simulink model "new_my_brake_system"  (R2024a)
settings: Solver=ode45  StartTime=0  StopTime=2000  FixedStep=.001  RelTol=1e-3  EnableMultiTasking=on
model workspace (MAT data in the model file):
  J = 0.226199211484
  Kt = 174.53
  Ts_verif : Simulink.Parameter (value not decoded)
  angle_init = 15
  angle_open = 85
  c = 8.89069171842
  fall_end_angle : Simulink.Parameter (value not decoded)
  fall_start_angle : Simulink.Parameter (value not decoded)
  input_delay = 0.00986306560803
  k = 19.1559540807
  rise_end_angle : Simulink.Parameter (value not decoded)
  rise_start_angle : Simulink.Parameter (value not decoded)
  vv_fall_time_max : Simulink.Parameter (value not decoded)
  vv_fall_time_min : Simulink.Parameter (value not decoded)
  vv_rise_time_max : Simulink.Parameter (value not decoded)
  vv_rise_time_min : Simulink.Parameter (value not decoded)
(part 2 of 2)

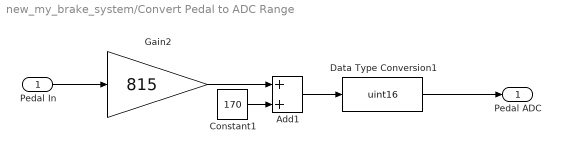
== system new_my_brake_system/Convert Pedal to ADC Range ==
  Pedal In : Inport
  Add1 : Sum
  Constant1 : Constant  Value=170
  Data Type Conversion1 : DataTypeConversion  OutDataTypeStr=uint16  SaturateOnIntegerOverflow=off  RndMeth=Floor
  Gain2 : Gain  Gain=815
  Pedal ADC : Outport  VectorParamsAs1DForOutWhenUnconnected=off
  wires:
  Gain2/1 -> Add1/1
  Constant1/1 -> Add1/2
  Data Type Conversion1/1 -> Pedal ADC/1
  Add1/1 -> Data Type Conversion1/1
  Pedal In/1 -> Gain2/1

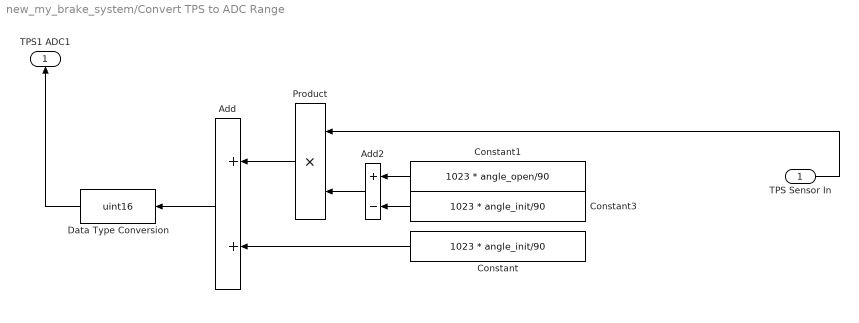
== system new_my_brake_system/Convert TPS to ADC Range ==
  TPS Sensor In : Inport
  Add : Sum
  Add2 : Sum  Inputs=+-
  Constant : Constant  Value=1023 * angle_init/90
  Constant1 : Constant  Value=1023 * angle_open/90
  Constant3 : Constant  Value=1023 * angle_init/90
  Data Type Conversion : DataTypeConversion  OutDataTypeStr=uint16  SaturateOnIntegerOverflow=off  RndMeth=Floor
  Product : Product
  TPS1 ADC1 : Outport  VectorParamsAs1DForOutWhenUnconnected=off
  wires:
  Product/1 -> Add/1
  Constant/1 -> Add/2
  Add/1 -> Data Type Conversion/1
  Data Type Conversion/1 -> TPS1 ADC1/1
  Add2/1 -> Product/2
  Constant1/1 -> Add2/1
  Constant3/1 -> Add2/2
  TPS Sensor In/1 -> Product/1

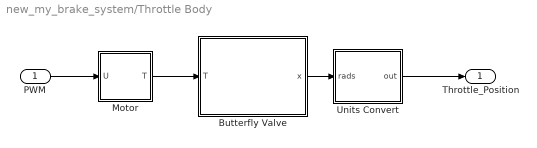
== system new_my_brake_system/Throttle Body ==
  PWM : Inport
  Butterfly Valve : Subsystem  mask{var_J=J, var_D=c, var_K=k, angle_init=angle_init, angle_open=angle_open}
      mask prompts: var_J "Inertia:"; var_D "Damping:"; var_K "Stiffness:"; angle_init "Resting Angle:"; angle_open "Open Angle:"
  Motor : Subsystem
  Units Convert : Subsystem
  Throttle_Position : Outport  VectorParamsAs1DForOutWhenUnconnected=off
  wires:
  PWM/1 -> Motor/1(U)
  Motor/1(T) -> Butterfly Valve/1(T)
  Units Convert/1(out) -> Throttle_Position/1
  Butterfly Valve/1(x) -> Units Convert/1(rads)

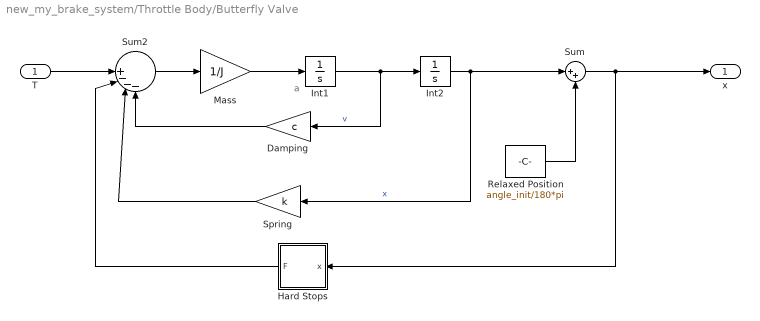
== system new_my_brake_system/Throttle Body/Butterfly Valve ==
  note: a
  T : Inport
  Damping : Gain  Gain=c  SaturateOnIntegerOverflow=on  OutDataTypeStr=Inherit: Same as input  ParamDataTypeStr=Inherit: Same as input
  Hard Stops : Subsystem  mask{H=angle_open/180*pi, K=2.86e5, L=angle_init/180*pi}
      mask prompts: H "Upper Limit:"; K "Stiffness:"; L "Lower Limit:"
  Int1 : Integrator
  Int2 : Integrator
  Mass : Gain  Gain=1/J  SaturateOnIntegerOverflow=on  OutDataTypeStr=Inherit: Same as input  ParamDataTypeStr=Inherit: Same as input
  Relaxed Position : Constant  Value=angle_init/180*pi
  Spring : Gain  Gain=k  SaturateOnIntegerOverflow=on  OutDataTypeStr=Inherit: Same as input  ParamDataTypeStr=Inherit: Same as input
  Sum : Sum  Inputs=|++  InputSameDT=on  SaturateOnIntegerOverflow=on  OutDataTypeStr=Inherit: Same as first input
  Sum2 : Sum  Inputs=|||+---  InputSameDT=on  SaturateOnIntegerOverflow=on  OutDataTypeStr=Inherit: Same as first input
  x : Outport  VectorParamsAs1DForOutWhenUnconnected=off
  wires:
  Hard Stops/1(F) -> Sum2/2
  Spring/1 -> Sum2/3
  Int2/1 -> Spring/1, Sum/1  "x"
  Relaxed Position/1 -> Sum/2
  Sum2/1 -> Mass/1
  T/1 -> Sum2/1
  Mass/1 -> Int1/1
  Int1/1 -> Damping/1, Int2/1  "v"
  Damping/1 -> Sum2/4
  Sum/1 -> x/1, Hard Stops/1(x)

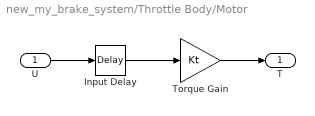
== system new_my_brake_system/Throttle Body/Motor ==
  U : Inport
  Input Delay : TransportDelay  DelayTime=input_delay
  Torque Gain : Gain  Gain=Kt  SaturateOnIntegerOverflow=on  OutDataTypeStr=Inherit: Same as input  ParamDataTypeStr=Inherit: Same as input
  T : Outport  VectorParamsAs1DForOutWhenUnconnected=off
  wires:
  U/1 -> Input Delay/1
  Torque Gain/1 -> T/1
  Input Delay/1 -> Torque Gain/1

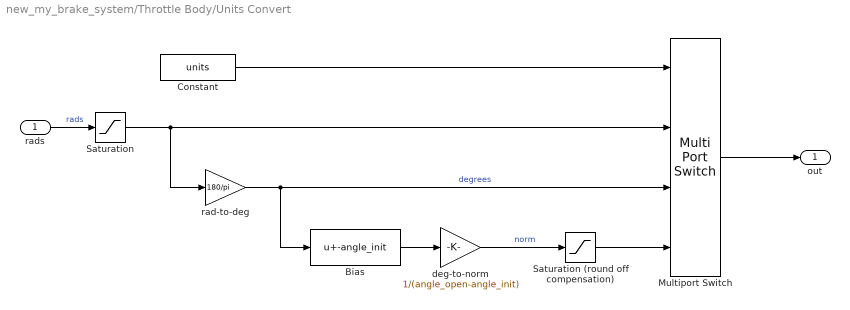
== system new_my_brake_system/Throttle Body/Units Convert ==
  rads : Inport
  Bias : Bias  Bias=-angle_init  SaturateOnIntegerOverflow=off
  Constant : Constant  Value=units
  Multiport Switch : MultiPortSwitch  SaturateOnIntegerOverflow=off  InputSameDT=off
  Saturation : Saturate  UpperLimit=pi/2  LowerLimit=0.0
  Saturation (round off compensation) : Saturate  UpperLimit=1.0  LowerLimit=0.0
  deg-to-norm : Gain  Gain=1/(angle_open-angle_init)
      settings: AttributesFormatString=%<Gain>
  rad-to-deg : Gain  Gain=180/pi
  out : Outport  VectorParamsAs1DForOutWhenUnconnected=off
  wires:
  Saturation/1 -> rad-to-deg/1, Multiport Switch/2
  Saturation (round off compensation)/1 -> Multiport Switch/4
  Bias/1 -> deg-to-norm/1
  deg-to-norm/1 -> Saturation (round off compensation)/1  "norm"
  Constant/1 -> Multiport Switch/1
  Multiport Switch/1 -> out/1
  rads/1 -> Saturation/1  "rads"
  rad-to-deg/1 -> Multiport Switch/3, Bias/1  "degrees"

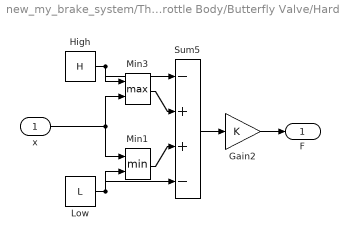
== system new_my_brake_system/Throttle Body/Butterfly Valve/Hard Stops ==
  x : Inport
  Gain2 : Gain  Gain=K  SaturateOnIntegerOverflow=on  OutDataTypeStr=Inherit: Same as input  ParamDataTypeStr=Inherit: Same as input
  High : Constant  Value=H
  Low : Constant  Value=L
  Min1 : MinMax  Inputs=2  InputSameDT=on  SaturateOnIntegerOverflow=on
  Min3 : MinMax  Function=max  Inputs=2  InputSameDT=on  SaturateOnIntegerOverflow=on
  Sum5 : Sum  Inputs=-+||+-  InputSameDT=on  SaturateOnIntegerOverflow=on  OutDataTypeStr=Inherit: Same as first input
  F : Outport  VectorParamsAs1DForOutWhenUnconnected=off
  wires:
  Gain2/1 -> F/1
  x/1 -> Min1/1, Min3/2
  Sum5/1 -> Gain2/1
  Low/1 -> Min1/2, Sum5/4
  High/1 -> Sum5/1, Min3/1
  Min3/1 -> Sum5/2
  Min1/1 -> Sum5/3
